simulink model "TST_EISGov_Governor"  (R2016b)
settings: Solver=FixedStepDiscrete  StartTime=0.0  StopTime=simTime  FixedStep=sampleTime  RelTol=1e-3
values from neighbouring files (symbols this model uses):
  testCase = 1    [initTST_EISGov_Governor_001.m]    (also in initTST_EISGov_Governor_002.m = 2; initTST_EISGov_Governor_003.m = 3; initTST_EISGov_Governor_004.m = 4; initTST_EISGov_Governor_005.m = 5)
libraries: simulink x43, UnitTest_Lib x36
(part 1 of 4)
settings Model: Creator=zhengjinyan  LastModifiedBy=zhengjinyan
settings DebuggingCC: SignalRangeChecking=error

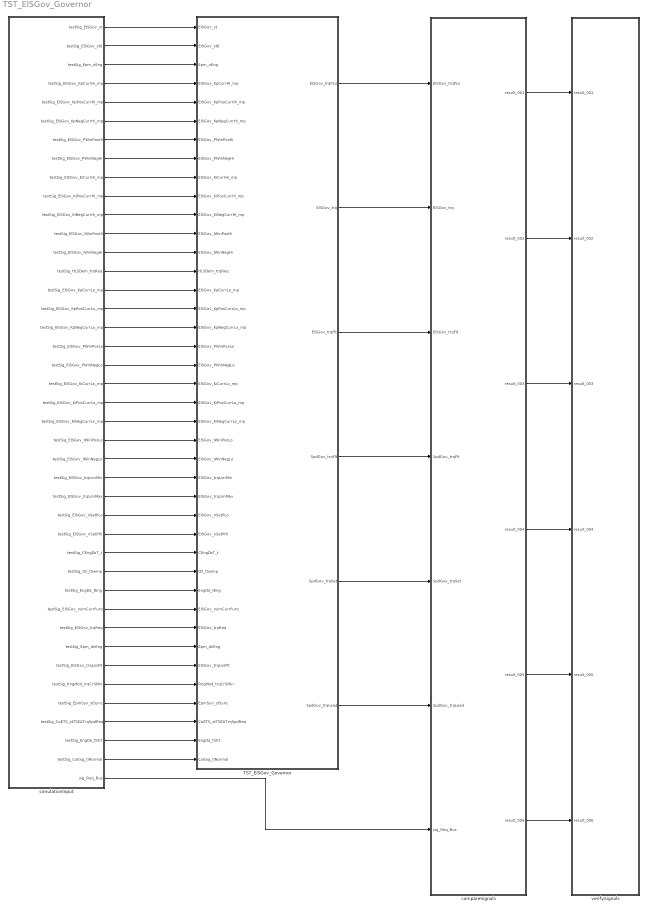
== system TST_EISGov_Governor ==
  TST_EISGov_Governor : Subsystem
  compareSignals : Subsystem
  simulationInput : Subsystem
  verifySignals : Subsystem
  wires:
  simulationInput/1(testSig_EISGov_st) -> TST_EISGov_Governor/1(EISGov_st)
  simulationInput/2(testSig_EISGov_st6) -> TST_EISGov_Governor/2(EISGov_st6)
  simulationInput/3(testSig_Epm_nEng) -> TST_EISGov_Governor/3(Epm_nEng)
  simulationInput/4(testSig_EISGov_KpCurrHi_mp) -> TST_EISGov_Governor/4(EISGov_KpCurrHi_mp)
  simulationInput/5(testSig_EISGov_KpPosCurrHi_mp) -> TST_EISGov_Governor/5(EISGov_KpPosCurrHi_mp)
  simulationInput/6(testSig_EISGov_KpNegCurrHi_mp) -> TST_EISGov_Governor/6(EISGov_KpNegCurrHi_mp)
  simulationInput/7(testSig_EISGov_PWinPosHi) -> TST_EISGov_Governor/7(EISGov_PWinPosHi)
  simulationInput/8(testSig_EISGov_PWinNegHi) -> TST_EISGov_Governor/8(EISGov_PWinNegHi)
  simulationInput/9(testSig_EISGov_KiCurrHi_mp) -> TST_EISGov_Governor/9(EISGov_KiCurrHi_mp)
  simulationInput/10(testSig_EISGov_KiPosCurrHi_mp) -> TST_EISGov_Governor/10(EISGov_KiPosCurrHi_mp)
  simulationInput/11(testSig_EISGov_KiNegCurrHi_mp) -> TST_EISGov_Governor/11(EISGov_KiNegCurrHi_mp)
  simulationInput/12(testSig_EISGov_IWinPosHi) -> TST_EISGov_Governor/12(EISGov_IWinPosHi)
  simulationInput/13(testSig_EISGov_IWinNegHi) -> TST_EISGov_Governor/13(EISGov_IWinNegHi)
  simulationInput/14(testSig_HLSDem_trqReq) -> TST_EISGov_Governor/14(HLSDem_trqReq)
  simulationInput/15(testSig_EISGov_KpCurrLo_mp) -> TST_EISGov_Governor/15(EISGov_KpCurrLo_mp)
  simulationInput/16(testSig_EISGov_KpPosCurrLo_mp) -> TST_EISGov_Governor/16(EISGov_KpPosCurrLo_mp)
  simulationInput/17(testSig_EISGov_KpNegCurrLo_mp) -> TST_EISGov_Governor/17(EISGov_KpNegCurrLo_mp)
  simulationInput/18(testSig_EISGov_PWinPosLo) -> TST_EISGov_Governor/18(EISGov_PWinPosLo)
  simulationInput/19(testSig_EISGov_PWinNegLo) -> TST_EISGov_Governor/19(EISGov_PWinNegLo)
  simulationInput/20(testSig_EISGov_KiCurrLo_mp) -> TST_EISGov_Governor/20(EISGov_KiCurrLo_mp)
  simulationInput/21(testSig_EISGov_KiPosCurrLo_mp) -> TST_EISGov_Governor/21(EISGov_KiPosCurrLo_mp)
  simulationInput/22(testSig_EISGov_KiNegCurrLo_mp) -> TST_EISGov_Governor/22(EISGov_KiNegCurrLo_mp)
  simulationInput/23(testSig_EISGov_IWinPosLo) -> TST_EISGov_Governor/23(EISGov_IWinPosLo)
  simulationInput/24(testSig_EISGov_IWinNegLo) -> TST_EISGov_Governor/24(EISGov_IWinNegLo)
  simulationInput/25(testSig_EISGov_trqLimMin) -> TST_EISGov_Governor/25(EISGov_trqLimMin)
  simulationInput/26(testSig_EISGov_trqLimMax) -> TST_EISGov_Governor/26(EISGov_trqLimMax)
  simulationInput/27(testSig_EISGov_nSetPLo) -> TST_EISGov_Governor/27(EISGov_nSetPLo)
  simulationInput/28(testSig_EISGov_nSetPHi) -> TST_EISGov_Governor/28(EISGov_nSetPHi)
  simulationInput/29(testSig_CEngDsT_t) -> TST_EISGov_Governor/29(CEngDsT_t)
  simulationInput/30(testSig_Oil_tSwmp) -> TST_EISGov_Governor/30(Oil_tSwmp)
  simulationInput/31(testSig_EngDa_tEng) -> TST_EISGov_Governor/31(EngDa_tEng)
  simulationInput/32(testSig_EISGov_numCurrFunc) -> TST_EISGov_Governor/32(EISGov_numCurrFunc)
  simulationInput/33(testSig_EISGov_trqReq) -> TST_EISGov_Governor/33(EISGov_trqReq)
  simulationInput/34(testSig_Epm_dnEng) -> TST_EISGov_Governor/34(Epm_dnEng)
  simulationInput/35(testSig_EISGov_trqLosFlt) -> TST_EISGov_Governor/35(EISGov_trqLosFlt)
  simulationInput/36(testSig_RngMod_trqCrSMin) -> TST_EISGov_Governor/36(RngMod_trqCrSMin)
  simulationInput/37(testSig_EpmSyn_stSync) -> TST_EISGov_Governor/37(EpmSyn_stSync)
  simulationInput/38(testSig_CoETS_stTSEATrqSpdReq) -> TST_EISGov_Governor/38(CoETS_stTSEATrqSpdReq)
  simulationInput/39(testSig_EngDa_tStrt) -> TST_EISGov_Governor/39(EngDa_tStrt)
  simulationInput/40(testSig_CoEng_tiNormal) -> TST_EISGov_Governor/40(CoEng_tiNormal)
  TST_EISGov_Governor/1(EISGov_trqPLo) -> compareSignals/1(EISGov_trqPLo)
  TST_EISGov_Governor/2(EISGov_trq) -> compareSignals/2(EISGov_trq)
  TST_EISGov_Governor/3(EISGov_trqFlt) -> compareSignals/3(EISGov_trqFlt)
  TST_EISGov_Governor/4(SpdGov_trqFlt) -> compareSignals/4(SpdGov_trqFlt)
  TST_EISGov_Governor/5(SpdGov_trqSet) -> compareSignals/5(SpdGov_trqSet)
  TST_EISGov_Governor/6(SpdGov_trqLead) -> compareSignals/6(SpdGov_trqLead)
  simulationInput/41(sig_Req_Bus) -> compareSignals/7(sig_Req_Bus)
  compareSignals/1(result_001) -> verifySignals/1(result_001)
  compareSignals/2(result_002) -> verifySignals/2(result_002)
  compareSignals/3(result_003) -> verifySignals/3(result_003)
  compareSignals/4(result_004) -> verifySignals/4(result_004)
  compareSignals/5(result_005) -> verifySignals/5(result_005)
  compareSignals/6(result_006) -> verifySignals/6(result_006)

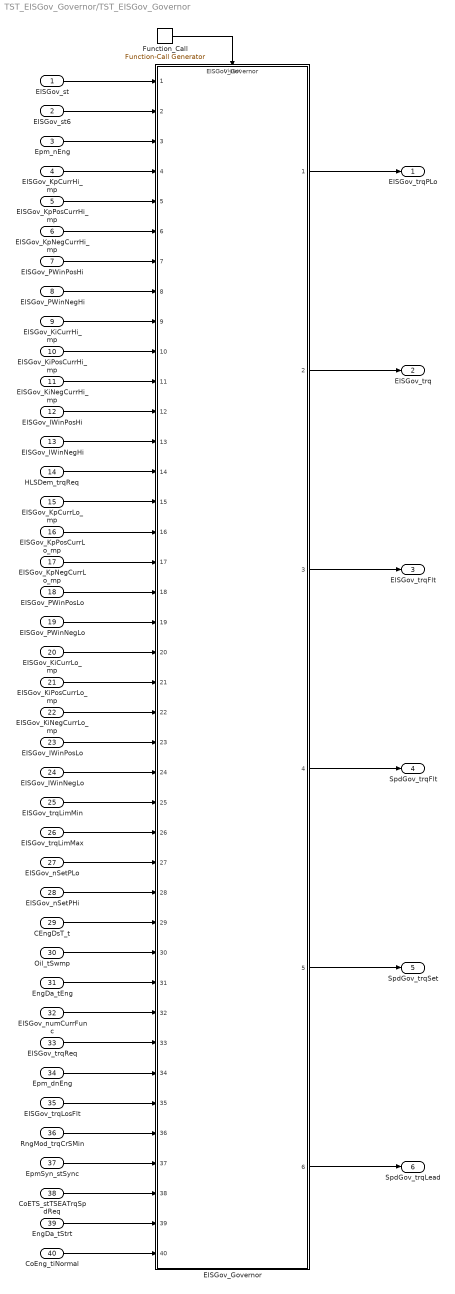
== system TST_EISGov_Governor/TST_EISGov_Governor ==
  EISGov_st : Inport
  EISGov_st6 : Inport  Port=2
  Epm_nEng : Inport  Port=3
  EISGov_KpCurrHi_mp : Inport  Port=4
  EISGov_KpPosCurrHi_mp : Inport  Port=5
  EISGov_KpNegCurrHi_mp : Inport  Port=6
  EISGov_PWinPosHi : Inport  Port=7
  EISGov_PWinNegHi : Inport  Port=8
  EISGov_KiCurrHi_mp : Inport  Port=9
  EISGov_KiPosCurrHi_mp : Inport  Port=10
  EISGov_KiNegCurrHi_mp : Inport  Port=11
  EISGov_IWinPosHi : Inport  Port=12
  EISGov_IWinNegHi : Inport  Port=13
  HLSDem_trqReq : Inport  Port=14
  EISGov_KpCurrLo_mp : Inport  Port=15
  EISGov_KpPosCurrLo_mp : Inport  Port=16
  EISGov_KpNegCurrLo_mp : Inport  Port=17
  EISGov_PWinPosLo : Inport  Port=18
  EISGov_PWinNegLo : Inport  Port=19
  EISGov_KiCurrLo_mp : Inport  Port=20
  EISGov_KiPosCurrLo_mp : Inport  Port=21
  EISGov_KiNegCurrLo_mp : Inport  Port=22
  EISGov_IWinPosLo : Inport  Port=23
  EISGov_IWinNegLo : Inport  Port=24
  EISGov_trqLimMin : Inport  Port=25
  EISGov_trqLimMax : Inport  Port=26
  EISGov_nSetPLo : Inport  Port=27
  EISGov_nSetPHi : Inport  Port=28
  CEngDsT_t : Inport  Port=29
  Oil_tSwmp : Inport  Port=30
  EngDa_tEng : Inport  Port=31
  EISGov_numCurrFunc : Inport  Port=32
  EISGov_trqReq : Inport  Port=33
  Epm_dnEng : Inport  Port=34
  EISGov_trqLosFlt : Inport  Port=35
  RngMod_trqCrSMin : Inport  Port=36
  EpmSyn_stSync : Inport  Port=37
  CoETS_stTSEATrqSpdReq : Inport  Port=38
  EngDa_tStrt : Inport  Port=39
  CoEng_tiNormal : Inport  Port=40
  EISGov_Governor : ModelReference  ModelNameDialog=EISGov_Governor  SimulationMode=Normal  ModelReferenceVersion=1.324  TriggerPortName=function  TriggerPortTriggerType=function-call  TriggerPortStatesWhenEnabling=held
  Function_Call : simulink/Ports & Subsystems/Function-Call Generator  sample_time=sampleTime  numberOfIterations=1
  EISGov_trqPLo : Outport
  EISGov_trq : Outport  Port=2
  EISGov_trqFlt : Outport  Port=3
  SpdGov_trqFlt : Outport  Port=4
  SpdGov_trqSet : Outport  Port=5
  SpdGov_trqLead : Outport  Port=6
  wires:
  Function_Call/1 -> EISGov_Governor/Trigger
  EISGov_st/1 -> EISGov_Governor/1
  EISGov_st6/1 -> EISGov_Governor/2
  Epm_nEng/1 -> EISGov_Governor/3
  EISGov_KpCurrHi_mp/1 -> EISGov_Governor/4
  EISGov_KpPosCurrHi_mp/1 -> EISGov_Governor/5
  EISGov_KpNegCurrHi_mp/1 -> EISGov_Governor/6
  EISGov_PWinPosHi/1 -> EISGov_Governor/7
  EISGov_PWinNegHi/1 -> EISGov_Governor/8
  EISGov_KiCurrHi_mp/1 -> EISGov_Governor/9
  EISGov_KiPosCurrHi_mp/1 -> EISGov_Governor/10
  EISGov_KiNegCurrHi_mp/1 -> EISGov_Governor/11
  EISGov_IWinPosHi/1 -> EISGov_Governor/12
  EISGov_IWinNegHi/1 -> EISGov_Governor/13
  HLSDem_trqReq/1 -> EISGov_Governor/14
  EISGov_KpCurrLo_mp/1 -> EISGov_Governor/15
  EISGov_KpPosCurrLo_mp/1 -> EISGov_Governor/16
  EISGov_KpNegCurrLo_mp/1 -> EISGov_Governor/17
  EISGov_PWinPosLo/1 -> EISGov_Governor/18
  EISGov_PWinNegLo/1 -> EISGov_Governor/19
  EISGov_KiCurrLo_mp/1 -> EISGov_Governor/20
  EISGov_KiPosCurrLo_mp/1 -> EISGov_Governor/21
  EISGov_KiNegCurrLo_mp/1 -> EISGov_Governor/22
  EISGov_IWinPosLo/1 -> EISGov_Governor/23
  EISGov_IWinNegLo/1 -> EISGov_Governor/24
  EISGov_trqLimMin/1 -> EISGov_Governor/25
  EISGov_trqLimMax/1 -> EISGov_Governor/26
  EISGov_nSetPLo/1 -> EISGov_Governor/27
  EISGov_nSetPHi/1 -> EISGov_Governor/28
  CEngDsT_t/1 -> EISGov_Governor/29
  Oil_tSwmp/1 -> EISGov_Governor/30
  EngDa_tEng/1 -> EISGov_Governor/31
  EISGov_numCurrFunc/1 -> EISGov_Governor/32
  EISGov_trqReq/1 -> EISGov_Governor/33
  Epm_dnEng/1 -> EISGov_Governor/34
  EISGov_trqLosFlt/1 -> EISGov_Governor/35
  RngMod_trqCrSMin/1 -> EISGov_Governor/36
  EpmSyn_stSync/1 -> EISGov_Governor/37
  CoETS_stTSEATrqSpdReq/1 -> EISGov_Governor/38
  EngDa_tStrt/1 -> EISGov_Governor/39
  CoEng_tiNormal/1 -> EISGov_Governor/40
  EISGov_Governor/1 -> EISGov_trqPLo/1
  EISGov_Governor/2 -> EISGov_trq/1
  EISGov_Governor/3 -> EISGov_trqFlt/1
  EISGov_Governor/4 -> SpdGov_trqFlt/1
  EISGov_Governor/5 -> SpdGov_trqSet/1
  EISGov_Governor/6 -> SpdGov_trqLead/1

== system TST_EISGov_Governor/compareSignals ==
  EISGov_trqPLo : Inport
  EISGov_trq : Inport  Port=2
  EISGov_trqFlt : Inport  Port=3
  SpdGov_trqFlt : Inport  Port=4
  SpdGov_trqSet : Inport  Port=5
  SpdGov_trqLead : Inport  Port=6
  sig_Req_Bus : Inport  Port=7
  BC : BusCreator  Inputs=6
  CTC_001 : simulink/Logic and Bit Operations/Compare To Constant  relop===  const=1  OutDataTypeStr=boolean
  CTC_002 : simulink/Logic and Bit Operations/Compare To Constant  relop===  const=2  OutDataTypeStr=boolean
  CTC_003 : simulink/Logic and Bit Operations/Compare To Constant  relop===  const=3  OutDataTypeStr=boolean
  CTC_004 : simulink/Logic and Bit Operations/Compare To Constant  relop===  const=4  OutDataTypeStr=boolean
  CTC_005 : simulink/Logic and Bit Operations/Compare To Constant  relop===  const=5  OutDataTypeStr=boolean
  CTC_006 : simulink/Logic and Bit Operations/Compare To Constant  relop===  const=6  OutDataTypeStr=boolean
  Requirement_001 : Subsystem
  Requirement_002 : Subsystem
  Requirement_003 : Subsystem
  Requirement_004 : Subsystem
  Requirement_005 : Subsystem
  Requirement_006 : Subsystem
  TC_001 : Constant  Value=testCase
  TC_002 : Constant  Value=testCase
  TC_003 : Constant  Value=testCase
  TC_004 : Constant  Value=testCase
  TC_005 : Constant  Value=testCase
  TC_006 : Constant  Value=testCase
  result_001 : Outport
  result_002 : Outport  Port=2
  result_003 : Outport  Port=3
  result_004 : Outport  Port=4
  result_005 : Outport  Port=5
  result_006 : Outport  Port=6
  wires:
  EISGov_trqPLo/1 -> BC/1  "EISGov_trqPLo"
  EISGov_trq/1 -> BC/2  "EISGov_trq"
  EISGov_trqFlt/1 -> BC/3  "EISGov_trqFlt"
  SpdGov_trqFlt/1 -> BC/4  "SpdGov_trqFlt"
  SpdGov_trqSet/1 -> BC/5  "SpdGov_trqSet"
  SpdGov_trqLead/1 -> BC/6  "SpdGov_trqLead"
  TC_001/1 -> CTC_001/1
  CTC_001/1 -> Requirement_001/Enable
  sig_Req_Bus/1 -> Requirement_001/2(sig_Req_Bus), Requirement_002/2(sig_Req_Bus), Requirement_003/2(sig_Req_Bus), Requirement_004/2(sig_Req_Bus), Requirement_005/2(sig_Req_Bus), Requirement_006/2(sig_Req_Bus)
  BC/1 -> Requirement_001/1(sig_Result_Bus), Requirement_002/1(sig_Result_Bus), Requirement_003/1(sig_Result_Bus), Requirement_004/1(sig_Result_Bus), Requirement_005/1(sig_Result_Bus), Requirement_006/1(sig_Result_Bus)
  Requirement_001/1(result) -> result_001/1
  TC_002/1 -> CTC_002/1
  CTC_002/1 -> Requirement_002/Enable
  Requirement_002/1(result) -> result_002/1
  TC_003/1 -> CTC_003/1
  CTC_003/1 -> Requirement_003/Enable
  Requirement_003/1(result) -> result_003/1
  TC_004/1 -> CTC_004/1
  CTC_004/1 -> Requirement_004/Enable
  Requirement_004/1(result) -> result_004/1
  TC_005/1 -> CTC_005/1
  CTC_005/1 -> Requirement_005/Enable
  Requirement_005/1(result) -> result_005/1
  TC_006/1 -> CTC_006/1
  CTC_006/1 -> Requirement_006/Enable
  Requirement_006/1(result) -> result_006/1

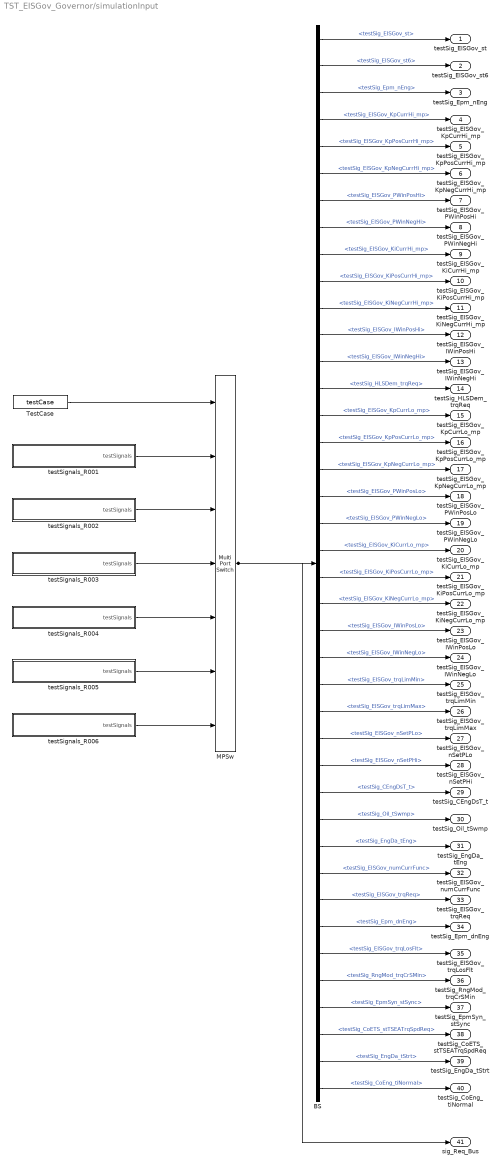
== system TST_EISGov_Governor/simulationInput ==
  BS : BusSelector  OutputSignals=testSig_EISGov_st,testSig_EISGov_st6,testSig_Epm_nEng,testSig_EISGov_KpCurrHi_mp,testSig_EISGov_KpPosCurrHi_mp,testSig_EISGov_KpNegCurrHi_mp,testSig_EISGov_PWinPosHi,testSig_EISGov_PWinNegHi,testSig_EISGov_KiCurrHi_mp,testSig_EISGov_KiPosCurrHi_mp,testSig_EISGov_KiNegCurrHi_mp,testSig_EISGov_IWinPosHi,testSig_EISGov_IWinNegHi,testSig_HLSDem_trqReq,testSig_EISGov_KpCurrLo_mp,testSig_EISGov_KpPosCurrLo_mp,testSig_EISGov_KpNegCurrLo_mp,testSig_EISGov_PWinPosLo,testSig_EISGov_PWinNegLo,testSig_EISGov_KiCurrLo_mp,testSig_EISGov_KiPosCurrLo_mp,testSig_EISGov_KiNegCurrLo_mp,testSig_EISGov_IWinPosLo,testSig_EISGov_IWinNegLo,testSig_EISGov_trqLimMin,testSig_EISGov_trqLimMax,testSig_EISGov_nSetPLo,testSig_EISGov_nSetPHi,testSig_CEngDsT_t,testSig_Oil_tSwmp,testSig_EngDa_tEng,testSig_EISGov_numCurrFunc,testSig_EISGov_trqReq,testSig_Epm_dnEng,testSig_EISGov_trqLosFlt,testSig_RngMod_trqCrSMin,testSig_EpmSyn_stSync,testSig_CoETS_stTSEATrqSpdReq,testSig_EngDa_tStrt,testSig_CoEng_tiNormal
  MPSw : MultiPortSwitch  Inputs=6  SaturateOnIntegerOverflow=on  InputSameDT=on
  TestCase : Constant  Value=testCase
  testSignals_R001 : Subsystem
  testSignals_R002 : Subsystem
  testSignals_R003 : Subsystem
  testSignals_R004 : Subsystem
  testSignals_R005 : Subsystem
  testSignals_R006 : Subsystem
  testSig_EISGov_st : Outport
  testSig_EISGov_st6 : Outport  Port=2
  testSig_Epm_nEng : Outport  Port=3
  testSig_EISGov_KpCurrHi_mp : Outport  Port=4
  testSig_EISGov_KpPosCurrHi_mp : Outport  Port=5
  testSig_EISGov_KpNegCurrHi_mp : Outport  Port=6
  testSig_EISGov_PWinPosHi : Outport  Port=7
  testSig_EISGov_PWinNegHi : Outport  Port=8
  testSig_EISGov_KiCurrHi_mp : Outport  Port=9
  testSig_EISGov_KiPosCurrHi_mp : Outport  Port=10
  testSig_EISGov_KiNegCurrHi_mp : Outport  Port=11
  testSig_EISGov_IWinPosHi : Outport  Port=12
  testSig_EISGov_IWinNegHi : Outport  Port=13
  testSig_HLSDem_trqReq : Outport  Port=14
  testSig_EISGov_KpCurrLo_mp : Outport  Port=15
  testSig_EISGov_KpPosCurrLo_mp : Outport  Port=16
  testSig_EISGov_KpNegCurrLo_mp : Outport  Port=17
  testSig_EISGov_PWinPosLo : Outport  Port=18
  testSig_EISGov_PWinNegLo : Outport  Port=19
  testSig_EISGov_KiCurrLo_mp : Outport  Port=20
  testSig_EISGov_KiPosCurrLo_mp : Outport  Port=21
  testSig_EISGov_KiNegCurrLo_mp : Outport  Port=22
  testSig_EISGov_IWinPosLo : Outport  Port=23
  testSig_EISGov_IWinNegLo : Outport  Port=24
  testSig_EISGov_trqLimMin : Outport  Port=25
  testSig_EISGov_trqLimMax : Outport  Port=26
  testSig_EISGov_nSetPLo : Outport  Port=27
  testSig_EISGov_nSetPHi : Outport  Port=28
  testSig_CEngDsT_t : Outport  Port=29
  testSig_Oil_tSwmp : Outport  Port=30
  testSig_EngDa_tEng : Outport  Port=31
  testSig_EISGov_numCurrFunc : Outport  Port=32
  testSig_EISGov_trqReq : Outport  Port=33
  testSig_Epm_dnEng : Outport  Port=34
  testSig_EISGov_trqLosFlt : Outport  Port=35
  testSig_RngMod_trqCrSMin : Outport  Port=36
  testSig_EpmSyn_stSync : Outport  Port=37
  testSig_CoETS_stTSEATrqSpdReq : Outport  Port=38
  testSig_EngDa_tStrt : Outport  Port=39
  testSig_CoEng_tiNormal : Outport  Port=40
  sig_Req_Bus : Outport  Port=41
  wires:
  BS/1 -> testSig_EISGov_st/1  "<testSig_EISGov_st>"
  BS/2 -> testSig_EISGov_st6/1  "<testSig_EISGov_st6>"
  BS/3 -> testSig_Epm_nEng/1  "<testSig_Epm_nEng>"
  BS/4 -> testSig_EISGov_KpCurrHi_mp/1  "<testSig_EISGov_KpCurrHi_mp>"
  BS/5 -> testSig_EISGov_KpPosCurrHi_mp/1  "<testSig_EISGov_KpPosCurrHi_mp>"
  BS/6 -> testSig_EISGov_KpNegCurrHi_mp/1  "<testSig_EISGov_KpNegCurrHi_mp>"
  BS/7 -> testSig_EISGov_PWinPosHi/1  "<testSig_EISGov_PWinPosHi>"
  BS/8 -> testSig_EISGov_PWinNegHi/1  "<testSig_EISGov_PWinNegHi>"
  BS/9 -> testSig_EISGov_KiCurrHi_mp/1  "<testSig_EISGov_KiCurrHi_mp>"
  BS/10 -> testSig_EISGov_KiPosCurrHi_mp/1  "<testSig_EISGov_KiPosCurrHi_mp>"
  BS/11 -> testSig_EISGov_KiNegCurrHi_mp/1  "<testSig_EISGov_KiNegCurrHi_mp>"
  BS/12 -> testSig_EISGov_IWinPosHi/1  "<testSig_EISGov_IWinPosHi>"
  BS/13 -> testSig_EISGov_IWinNegHi/1  "<testSig_EISGov_IWinNegHi>"
  BS/14 -> testSig_HLSDem_trqReq/1  "<testSig_HLSDem_trqReq>"
  BS/15 -> testSig_EISGov_KpCurrLo_mp/1  "<testSig_EISGov_KpCurrLo_mp>"
  BS/16 -> testSig_EISGov_KpPosCurrLo_mp/1  "<testSig_EISGov_KpPosCurrLo_mp>"
  BS/17 -> testSig_EISGov_KpNegCurrLo_mp/1  "<testSig_EISGov_KpNegCurrLo_mp>"
  BS/18 -> testSig_EISGov_PWinPosLo/1  "<testSig_EISGov_PWinPosLo>"
  BS/19 -> testSig_EISGov_PWinNegLo/1  "<testSig_EISGov_PWinNegLo>"
  BS/20 -> testSig_EISGov_KiCurrLo_mp/1  "<testSig_EISGov_KiCurrLo_mp>"
  BS/21 -> testSig_EISGov_KiPosCurrLo_mp/1  "<testSig_EISGov_KiPosCurrLo_mp>"
  BS/22 -> testSig_EISGov_KiNegCurrLo_mp/1  "<testSig_EISGov_KiNegCurrLo_mp>"
  BS/23 -> testSig_EISGov_IWinPosLo/1  "<testSig_EISGov_IWinPosLo>"
  BS/24 -> testSig_EISGov_IWinNegLo/1  "<testSig_EISGov_IWinNegLo>"
  BS/25 -> testSig_EISGov_trqLimMin/1  "<testSig_EISGov_trqLimMin>"
  BS/26 -> testSig_EISGov_trqLimMax/1  "<testSig_EISGov_trqLimMax>"
  BS/27 -> testSig_EISGov_nSetPLo/1  "<testSig_EISGov_nSetPLo>"
  BS/28 -> testSig_EISGov_nSetPHi/1  "<testSig_EISGov_nSetPHi>"
  BS/29 -> testSig_CEngDsT_t/1  "<testSig_CEngDsT_t>"
  BS/30 -> testSig_Oil_tSwmp/1  "<testSig_Oil_tSwmp>"
  BS/31 -> testSig_EngDa_tEng/1  "<testSig_EngDa_tEng>"
  BS/32 -> testSig_EISGov_numCurrFunc/1  "<testSig_EISGov_numCurrFunc>"
  BS/33 -> testSig_EISGov_trqReq/1  "<testSig_EISGov_trqReq>"
  BS/34 -> testSig_Epm_dnEng/1  "<testSig_Epm_dnEng>"
  BS/35 -> testSig_EISGov_trqLosFlt/1  "<testSig_EISGov_trqLosFlt>"
  BS/36 -> testSig_RngMod_trqCrSMin/1  "<testSig_RngMod_trqCrSMin>"
  BS/37 -> testSig_EpmSyn_stSync/1  "<testSig_EpmSyn_stSync>"
  BS/38 -> testSig_CoETS_stTSEATrqSpdReq/1  "<testSig_CoETS_stTSEATrqSpdReq>"
  BS/39 -> testSig_EngDa_tStrt/1  "<testSig_EngDa_tStrt>"
  BS/40 -> testSig_CoEng_tiNormal/1  "<testSig_CoEng_tiNormal>"
  MPSw/1 -> BS/1, sig_Req_Bus/1
  TestCase/1 -> MPSw/1
  testSignals_R001/1(testSignals) -> MPSw/2
  testSignals_R002/1(testSignals) -> MPSw/3
  testSignals_R003/1(testSignals) -> MPSw/4
  testSignals_R004/1(testSignals) -> MPSw/5
  testSignals_R005/1(testSignals) -> MPSw/6
  testSignals_R006/1(testSignals) -> MPSw/7

== system TST_EISGov_Governor/verifySignals ==
  result_001 : Inport
  result_002 : Inport  Port=2
  result_003 : Inport  Port=3
  result_004 : Inport  Port=4
  result_005 : Inport  Port=5
  result_006 : Inport  Port=6
  Assertion_001 : Assertion  Enabled=off
  Assertion_002 : Assertion  Enabled=off
  Assertion_003 : Assertion  Enabled=off
  Assertion_004 : Assertion  Enabled=off
  Assertion_005 : Assertion  Enabled=off
  Assertion_006 : Assertion  Enabled=off
  wires:
  result_001/1 -> Assertion_001/1
  result_002/1 -> Assertion_002/1
  result_003/1 -> Assertion_003/1
  result_004/1 -> Assertion_004/1
  result_005/1 -> Assertion_005/1
  result_006/1 -> Assertion_006/1

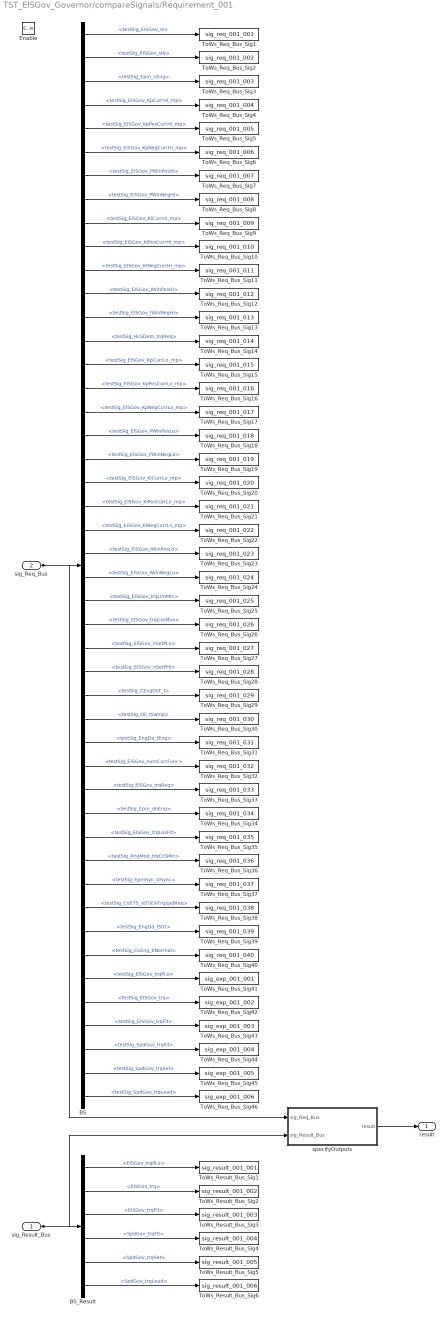
== system TST_EISGov_Governor/compareSignals/Requirement_001 ==
  sig_Result_Bus : Inport
  sig_Req_Bus : Inport  Port=2
  Enable : EnablePort
  BS : BusSelector  OutputSignals=testSig_EISGov_st,testSig_EISGov_st6,testSig_Epm_nEng,testSig_EISGov_KpCurrHi_mp,testSig_EISGov_KpPosCurrHi_mp,testSig_EISGov_KpNegCurrHi_mp,testSig_EISGov_PWinPosHi,testSig_EISGov_PWinNegHi,testSig_EISGov_KiCurrHi_mp,testSig_EISGov_KiPosCurrHi_mp,testSig_EISGov_KiNegCurrHi_mp,testSig_EISGov_IWinPosHi,testSig_EISGov_IWinNegHi,testSig_HLSDem_trqReq,testSig_EISGov_KpCurrLo_mp,testSig_EISGov_KpPosCurrLo_mp,testSig_EISGov_KpNegCurrLo_mp,testSig_EISGov_PWinPosLo,testSig_EISGov_PWinNegLo,testSig_EISGov_KiCurrLo_mp,testSig_EISGov_KiPosCurrLo_mp,testSig_EISGov_KiNegCurrLo_mp,testSig_EISGov_IWinPosLo,testSig_EISGov_IWinNegLo,testSig_EISGov_trqLimMin,testSig_EISGov_trqLimMax,testSig_EISGov_nSetPLo,testSig_EISGov_nSetPHi,testSig_CEngDsT_t,testSig_Oil_tSwmp,testSig_EngDa_tEng,testSig_EISGov_numCurrFunc,testSig_EISGov_trqReq,testSig_Epm_dnEng,testSig_EISGov_trqLosFlt,testSig_RngMod_trqCrSMin,testSig_EpmSyn_stSync,testSig_CoETS_stTSEATrqSpdReq,testSig_EngDa_tStrt,testSig_CoEng_tiNormal,testSig_EISGov_trqPLo,testSig_EISGov_trq,testSig_EISGov_trqFlt,testSig_SpdGov_trqFlt,testSig_SpdGov_trqSet,testSig_SpdGov_trqLead
  BS_Result : BusSelector  OutputSignals=EISGov_trqPLo,EISGov_trq,EISGov_trqFlt,SpdGov_trqFlt,SpdGov_trqSet,SpdGov_trqLead
  ToWs_Req_Bus_Sig1 : ToWorkspace  VariableName=sig_req_001_001  SaveFormat=Structure With Time
  ToWs_Req_Bus_Sig10 : ToWorkspace  VariableName=sig_req_001_010  SaveFormat=Structure With Time
  ToWs_Req_Bus_Sig11 : ToWorkspace  VariableName=sig_req_001_011  SaveFormat=Structure With Time
  ToWs_Req_Bus_Sig12 : ToWorkspace  VariableName=sig_req_001_012  SaveFormat=Structure With Time
  ToWs_Req_Bus_Sig13 : ToWorkspace  VariableName=sig_req_001_013  SaveFormat=Structure With Time
  ToWs_Req_Bus_Sig14 : ToWorkspace  VariableName=sig_req_001_014  SaveFormat=Structure With Time
  ToWs_Req_Bus_Sig15 : ToWorkspace  VariableName=sig_req_001_015  SaveFormat=Structure With Time
  ToWs_Req_Bus_Sig16 : ToWorkspace  VariableName=sig_req_001_016  SaveFormat=Structure With Time
  ToWs_Req_Bus_Sig17 : ToWorkspace  VariableName=sig_req_001_017  SaveFormat=Structure With Time
  ToWs_Req_Bus_Sig18 : ToWorkspace  VariableName=sig_req_001_018  SaveFormat=Structure With Time
  ToWs_Req_Bus_Sig19 : ToWorkspace  VariableName=sig_req_001_019  SaveFormat=Structure With Time
  ToWs_Req_Bus_Sig2 : ToWorkspace  VariableName=sig_req_001_002  SaveFormat=Structure With Time
  ToWs_Req_Bus_Sig20 : ToWorkspace  VariableName=sig_req_001_020  SaveFormat=Structure With Time
  ToWs_Req_Bus_Sig21 : ToWorkspace  VariableName=sig_req_001_021  SaveFormat=Structure With Time
  ToWs_Req_Bus_Sig22 : ToWorkspace  VariableName=sig_req_001_022  SaveFormat=Structure With Time
  ToWs_Req_Bus_Sig23 : ToWorkspace  VariableName=sig_req_001_023  SaveFormat=Structure With Time
  ToWs_Req_Bus_Sig24 : ToWorkspace  VariableName=sig_req_001_024  SaveFormat=Structure With Time
  ToWs_Req_Bus_Sig25 : ToWorkspace  VariableName=sig_req_001_025  SaveFormat=Structure With Time
  ToWs_Req_Bus_Sig26 : ToWorkspace  VariableName=sig_req_001_026  SaveFormat=Structure With Time
  ToWs_Req_Bus_Sig27 : ToWorkspace  VariableName=sig_req_001_027  SaveFormat=Structure With Time
  ToWs_Req_Bus_Sig28 : ToWorkspace  VariableName=sig_req_001_028  SaveFormat=Structure With Time
  ToWs_Req_Bus_Sig29 : ToWorkspace  VariableName=sig_req_001_029  SaveFormat=Structure With Time
  ToWs_Req_Bus_Sig3 : ToWorkspace  VariableName=sig_req_001_003  SaveFormat=Structure With Time
  ToWs_Req_Bus_Sig30 : ToWorkspace  VariableName=sig_req_001_030  SaveFormat=Structure With Time
  ToWs_Req_Bus_Sig31 : ToWorkspace  VariableName=sig_req_001_031  SaveFormat=Structure With Time
  ToWs_Req_Bus_Sig32 : ToWorkspace  VariableName=sig_req_001_032  SaveFormat=Structure With Time
  ToWs_Req_Bus_Sig33 : ToWorkspace  VariableName=sig_req_001_033  SaveFormat=Structure With Time
  ToWs_Req_Bus_Sig34 : ToWorkspace  VariableName=sig_req_001_034  SaveFormat=Structure With Time
  ToWs_Req_Bus_Sig35 : ToWorkspace  VariableName=sig_req_001_035  SaveFormat=Structure With Time
  ToWs_Req_Bus_Sig36 : ToWorkspace  VariableName=sig_req_001_036  SaveFormat=Structure With Time
  ToWs_Req_Bus_Sig37 : ToWorkspace  VariableName=sig_req_001_037  SaveFormat=Structure With Time
  ToWs_Req_Bus_Sig38 : ToWorkspace  VariableName=sig_req_001_038  SaveFormat=Structure With Time
  ToWs_Req_Bus_Sig39 : ToWorkspace  VariableName=sig_req_001_039  SaveFormat=Structure With Time
  ToWs_Req_Bus_Sig4 : ToWorkspace  VariableName=sig_req_001_004  SaveFormat=Structure With Time
  ToWs_Req_Bus_Sig40 : ToWorkspace  VariableName=sig_req_001_040  SaveFormat=Structure With Time
  ToWs_Req_Bus_Sig41 : ToWorkspace  VariableName=sig_exp_001_001  SaveFormat=Structure With Time
  ToWs_Req_Bus_Sig42 : ToWorkspace  VariableName=sig_exp_001_002  SaveFormat=Structure With Time
  ToWs_Req_Bus_Sig43 : ToWorkspace  VariableName=sig_exp_001_003  SaveFormat=Structure With Time
  ToWs_Req_Bus_Sig44 : ToWorkspace  VariableName=sig_exp_001_004  SaveFormat=Structure With Time
  ToWs_Req_Bus_Sig45 : ToWorkspace  VariableName=sig_exp_001_005  SaveFormat=Structure With Time
  ToWs_Req_Bus_Sig46 : ToWorkspace  VariableName=sig_exp_001_006  SaveFormat=Structure With Time
  ToWs_Req_Bus_Sig5 : ToWorkspace  VariableName=sig_req_001_005  SaveFormat=Structure With Time
  ToWs_Req_Bus_Sig6 : ToWorkspace  VariableName=sig_req_001_006  SaveFormat=Structure With Time
  ToWs_Req_Bus_Sig7 : ToWorkspace  VariableName=sig_req_001_007  SaveFormat=Structure With Time
  ToWs_Req_Bus_Sig8 : ToWorkspace  VariableName=sig_req_001_008  SaveFormat=Structure With Time
  ToWs_Req_Bus_Sig9 : ToWorkspace  VariableName=sig_req_001_009  SaveFormat=Structure With Time
  ToWs_Result_Bus_Sig1 : ToWorkspace  VariableName=sig_result_001_001  SaveFormat=Structure With Time
  ToWs_Result_Bus_Sig2 : ToWorkspace  VariableName=sig_result_001_002  SaveFormat=Structure With Time
  ToWs_Result_Bus_Sig3 : ToWorkspace  VariableName=sig_result_001_003  SaveFormat=Structure With Time
  ToWs_Result_Bus_Sig4 : ToWorkspace  VariableName=sig_result_001_004  SaveFormat=Structure With Time
  ToWs_Result_Bus_Sig5 : ToWorkspace  VariableName=sig_result_001_005  SaveFormat=Structure With Time
  ToWs_Result_Bus_Sig6 : ToWorkspace  VariableName=sig_result_001_006  SaveFormat=Structure With Time
  specifyOutputs : Subsystem
  result : Outport
  wires:
  sig_Req_Bus/1 -> BS/1, specifyOutputs/1(sig_Req_Bus)
  BS/1 -> ToWs_Req_Bus_Sig1/1  "<testSig_EISGov_st>"
  BS/2 -> ToWs_Req_Bus_Sig2/1  "<testSig_EISGov_st6>"
  BS/3 -> ToWs_Req_Bus_Sig3/1  "<testSig_Epm_nEng>"
  BS/4 -> ToWs_Req_Bus_Sig4/1  "<testSig_EISGov_KpCurrHi_mp>"
  BS/5 -> ToWs_Req_Bus_Sig5/1  "<testSig_EISGov_KpPosCurrHi_mp>"
  BS/6 -> ToWs_Req_Bus_Sig6/1  "<testSig_EISGov_KpNegCurrHi_mp>"
  BS/7 -> ToWs_Req_Bus_Sig7/1  "<testSig_EISGov_PWinPosHi>"
  BS/8 -> ToWs_Req_Bus_Sig8/1  "<testSig_EISGov_PWinNegHi>"
  BS/9 -> ToWs_Req_Bus_Sig9/1  "<testSig_EISGov_KiCurrHi_mp>"
  BS/10 -> ToWs_Req_Bus_Sig10/1  "<testSig_EISGov_KiPosCurrHi_mp>"
  BS/11 -> ToWs_Req_Bus_Sig11/1  "<testSig_EISGov_KiNegCurrHi_mp>"
  BS/12 -> ToWs_Req_Bus_Sig12/1  "<testSig_EISGov_IWinPosHi>"
  BS/13 -> ToWs_Req_Bus_Sig13/1  "<testSig_EISGov_IWinNegHi>"
  BS/14 -> ToWs_Req_Bus_Sig14/1  "<testSig_HLSDem_trqReq>"
  BS/15 -> ToWs_Req_Bus_Sig15/1  "<testSig_EISGov_KpCurrLo_mp>"
  BS/16 -> ToWs_Req_Bus_Sig16/1  "<testSig_EISGov_KpPosCurrLo_mp>"
  BS/17 -> ToWs_Req_Bus_Sig17/1  "<testSig_EISGov_KpNegCurrLo_mp>"
  BS/18 -> ToWs_Req_Bus_Sig18/1  "<testSig_EISGov_PWinPosLo>"
  BS/19 -> ToWs_Req_Bus_Sig19/1  "<testSig_EISGov_PWinNegLo>"
  BS/20 -> ToWs_Req_Bus_Sig20/1  "<testSig_EISGov_KiCurrLo_mp>"
  BS/21 -> ToWs_Req_Bus_Sig21/1  "<testSig_EISGov_KiPosCurrLo_mp>"
  BS/22 -> ToWs_Req_Bus_Sig22/1  "<testSig_EISGov_KiNegCurrLo_mp>"
  BS/23 -> ToWs_Req_Bus_Sig23/1  "<testSig_EISGov_IWinPosLo>"
  BS/24 -> ToWs_Req_Bus_Sig24/1  "<testSig_EISGov_IWinNegLo>"
  BS/25 -> ToWs_Req_Bus_Sig25/1  "<testSig_EISGov_trqLimMin>"
  BS/26 -> ToWs_Req_Bus_Sig26/1  "<testSig_EISGov_trqLimMax>"
  BS/27 -> ToWs_Req_Bus_Sig27/1  "<testSig_EISGov_nSetPLo>"
  BS/28 -> ToWs_Req_Bus_Sig28/1  "<testSig_EISGov_nSetPHi>"
  BS/29 -> ToWs_Req_Bus_Sig29/1  "<testSig_CEngDsT_t>"
  BS/30 -> ToWs_Req_Bus_Sig30/1  "<testSig_Oil_tSwmp>"
  BS/31 -> ToWs_Req_Bus_Sig31/1  "<testSig_EngDa_tEng>"
  BS/32 -> ToWs_Req_Bus_Sig32/1  "<testSig_EISGov_numCurrFunc>"
  BS/33 -> ToWs_Req_Bus_Sig33/1  "<testSig_EISGov_trqReq>"
  BS/34 -> ToWs_Req_Bus_Sig34/1  "<testSig_Epm_dnEng>"
  BS/35 -> ToWs_Req_Bus_Sig35/1  "<testSig_EISGov_trqLosFlt>"
  BS/36 -> ToWs_Req_Bus_Sig36/1  "<testSig_RngMod_trqCrSMin>"
  BS/37 -> ToWs_Req_Bus_Sig37/1  "<testSig_EpmSyn_stSync>"
  BS/38 -> ToWs_Req_Bus_Sig38/1  "<testSig_CoETS_stTSEATrqSpdReq>"
  BS/39 -> ToWs_Req_Bus_Sig39/1  "<testSig_EngDa_tStrt>"
  BS/40 -> ToWs_Req_Bus_Sig40/1  "<testSig_CoEng_tiNormal>"
  BS/41 -> ToWs_Req_Bus_Sig41/1  "<testSig_EISGov_trqPLo>"
  BS/42 -> ToWs_Req_Bus_Sig42/1  "<testSig_EISGov_trq>"
  BS/43 -> ToWs_Req_Bus_Sig43/1  "<testSig_EISGov_trqFlt>"
  BS/44 -> ToWs_Req_Bus_Sig44/1  "<testSig_SpdGov_trqFlt>"
  BS/45 -> ToWs_Req_Bus_Sig45/1  "<testSig_SpdGov_trqSet>"
  BS/46 -> ToWs_Req_Bus_Sig46/1  "<testSig_SpdGov_trqLead>"
  sig_Result_Bus/1 -> BS_Result/1, specifyOutputs/2(sig_Result_Bus)
  BS_Result/1 -> ToWs_Result_Bus_Sig1/1  "<EISGov_trqPLo>"
  BS_Result/2 -> ToWs_Result_Bus_Sig2/1  "<EISGov_trq>"
  BS_Result/3 -> ToWs_Result_Bus_Sig3/1  "<EISGov_trqFlt>"
  BS_Result/4 -> ToWs_Result_Bus_Sig4/1  "<SpdGov_trqFlt>"
  BS_Result/5 -> ToWs_Result_Bus_Sig5/1  "<SpdGov_trqSet>"
  BS_Result/6 -> ToWs_Result_Bus_Sig6/1  "<SpdGov_trqLead>"
  specifyOutputs/1(result) -> result/1

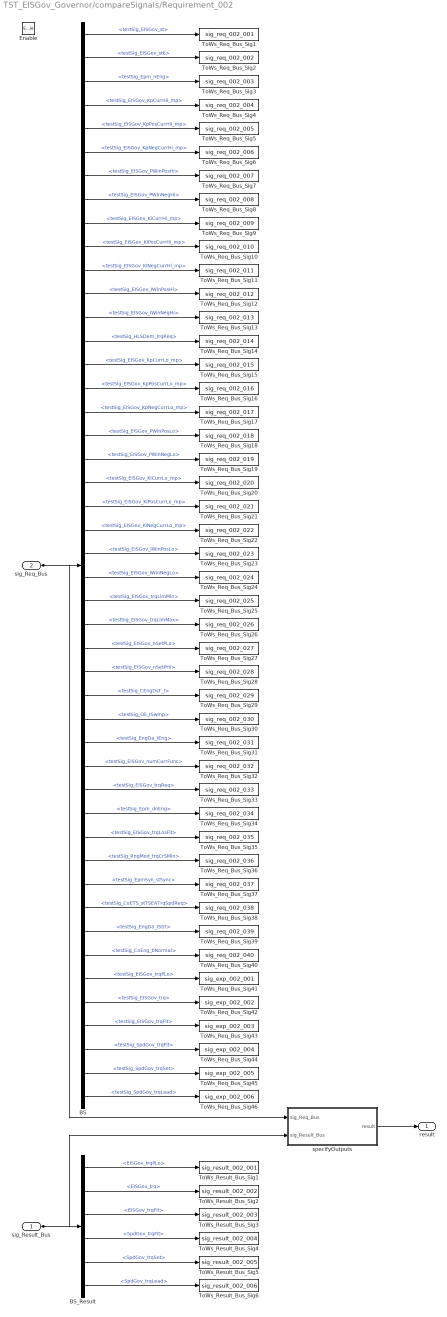
== system TST_EISGov_Governor/compareSignals/Requirement_002 ==
  sig_Result_Bus : Inport
  sig_Req_Bus : Inport  Port=2
  Enable : EnablePort
  BS : BusSelector  OutputSignals=testSig_EISGov_st,testSig_EISGov_st6,testSig_Epm_nEng,testSig_EISGov_KpCurrHi_mp,testSig_EISGov_KpPosCurrHi_mp,testSig_EISGov_KpNegCurrHi_mp,testSig_EISGov_PWinPosHi,testSig_EISGov_PWinNegHi,testSig_EISGov_KiCurrHi_mp,testSig_EISGov_KiPosCurrHi_mp,testSig_EISGov_KiNegCurrHi_mp,testSig_EISGov_IWinPosHi,testSig_EISGov_IWinNegHi,testSig_HLSDem_trqReq,testSig_EISGov_KpCurrLo_mp,testSig_EISGov_KpPosCurrLo_mp,testSig_EISGov_KpNegCurrLo_mp,testSig_EISGov_PWinPosLo,testSig_EISGov_PWinNegLo,testSig_EISGov_KiCurrLo_mp,testSig_EISGov_KiPosCurrLo_mp,testSig_EISGov_KiNegCurrLo_mp,testSig_EISGov_IWinPosLo,testSig_EISGov_IWinNegLo,testSig_EISGov_trqLimMin,testSig_EISGov_trqLimMax,testSig_EISGov_nSetPLo,testSig_EISGov_nSetPHi,testSig_CEngDsT_t,testSig_Oil_tSwmp,testSig_EngDa_tEng,testSig_EISGov_numCurrFunc,testSig_EISGov_trqReq,testSig_Epm_dnEng,testSig_EISGov_trqLosFlt,testSig_RngMod_trqCrSMin,testSig_EpmSyn_stSync,testSig_CoETS_stTSEATrqSpdReq,testSig_EngDa_tStrt,testSig_CoEng_tiNormal,testSig_EISGov_trqPLo,testSig_EISGov_trq,testSig_EISGov_trqFlt,testSig_SpdGov_trqFlt,testSig_SpdGov_trqSet,testSig_SpdGov_trqLead
  BS_Result : BusSelector  OutputSignals=EISGov_trqPLo,EISGov_trq,EISGov_trqFlt,SpdGov_trqFlt,SpdGov_trqSet,SpdGov_trqLead
  ToWs_Req_Bus_Sig1 : ToWorkspace  VariableName=sig_req_002_001  SaveFormat=Structure With Time
  ToWs_Req_Bus_Sig10 : ToWorkspace  VariableName=sig_req_002_010  SaveFormat=Structure With Time
  ToWs_Req_Bus_Sig11 : ToWorkspace  VariableName=sig_req_002_011  SaveFormat=Structure With Time
  ToWs_Req_Bus_Sig12 : ToWorkspace  VariableName=sig_req_002_012  SaveFormat=Structure With Time
  ToWs_Req_Bus_Sig13 : ToWorkspace  VariableName=sig_req_002_013  SaveFormat=Structure With Time
  ToWs_Req_Bus_Sig14 : ToWorkspace  VariableName=sig_req_002_014  SaveFormat=Structure With Time
  ToWs_Req_Bus_Sig15 : ToWorkspace  VariableName=sig_req_002_015  SaveFormat=Structure With Time
  ToWs_Req_Bus_Sig16 : ToWorkspace  VariableName=sig_req_002_016  SaveFormat=Structure With Time
  ToWs_Req_Bus_Sig17 : ToWorkspace  VariableName=sig_req_002_017  SaveFormat=Structure With Time
  ToWs_Req_Bus_Sig18 : ToWorkspace  VariableName=sig_req_002_018  SaveFormat=Structure With Time
  ToWs_Req_Bus_Sig19 : ToWorkspace  VariableName=sig_req_002_019  SaveFormat=Structure With Time
  ToWs_Req_Bus_Sig2 : ToWorkspace  VariableName=sig_req_002_002  SaveFormat=Structure With Time
  ToWs_Req_Bus_Sig20 : ToWorkspace  VariableName=sig_req_002_020  SaveFormat=Structure With Time
  ToWs_Req_Bus_Sig21 : ToWorkspace  VariableName=sig_req_002_021  SaveFormat=Structure With Time
  ToWs_Req_Bus_Sig22 : ToWorkspace  VariableName=sig_req_002_022  SaveFormat=Structure With Time
  ToWs_Req_Bus_Sig23 : ToWorkspace  VariableName=sig_req_002_023  SaveFormat=Structure With Time
  ToWs_Req_Bus_Sig24 : ToWorkspace  VariableName=sig_req_002_024  SaveFormat=Structure With Time
  ToWs_Req_Bus_Sig25 : ToWorkspace  VariableName=sig_req_002_025  SaveFormat=Structure With Time
  ToWs_Req_Bus_Sig26 : ToWorkspace  VariableName=sig_req_002_026  SaveFormat=Structure With Time
  ToWs_Req_Bus_Sig27 : ToWorkspace  VariableName=sig_req_002_027  SaveFormat=Structure With Time
  ToWs_Req_Bus_Sig28 : ToWorkspace  VariableName=sig_req_002_028  SaveFormat=Structure With Time
  ToWs_Req_Bus_Sig29 : ToWorkspace  VariableName=sig_req_002_029  SaveFormat=Structure With Time
  ToWs_Req_Bus_Sig3 : ToWorkspace  VariableName=sig_req_002_003  SaveFormat=Structure With Time
  ToWs_Req_Bus_Sig30 : ToWorkspace  VariableName=sig_req_002_030  SaveFormat=Structure With Time
  ToWs_Req_Bus_Sig31 : ToWorkspace  VariableName=sig_req_002_031  SaveFormat=Structure With Time
  ToWs_Req_Bus_Sig32 : ToWorkspace  VariableName=sig_req_002_032  SaveFormat=Structure With Time
  ToWs_Req_Bus_Sig33 : ToWorkspace  VariableName=sig_req_002_033  SaveFormat=Structure With Time
  ToWs_Req_Bus_Sig34 : ToWorkspace  VariableName=sig_req_002_034  SaveFormat=Structure With Time
  ToWs_Req_Bus_Sig35 : ToWorkspace  VariableName=sig_req_002_035  SaveFormat=Structure With Time
  ToWs_Req_Bus_Sig36 : ToWorkspace  VariableName=sig_req_002_036  SaveFormat=Structure With Time
  ToWs_Req_Bus_Sig37 : ToWorkspace  VariableName=sig_req_002_037  SaveFormat=Structure With Time
  ToWs_Req_Bus_Sig38 : ToWorkspace  VariableName=sig_req_002_038  SaveFormat=Structure With Time
  ToWs_Req_Bus_Sig39 : ToWorkspace  VariableName=sig_req_002_039  SaveFormat=Structure With Time
  ToWs_Req_Bus_Sig4 : ToWorkspace  VariableName=sig_req_002_004  SaveFormat=Structure With Time
  ToWs_Req_Bus_Sig40 : ToWorkspace  VariableName=sig_req_002_040  SaveFormat=Structure With Time
  ToWs_Req_Bus_Sig41 : ToWorkspace  VariableName=sig_exp_002_001  SaveFormat=Structure With Time
  ToWs_Req_Bus_Sig42 : ToWorkspace  VariableName=sig_exp_002_002  SaveFormat=Structure With Time
  ToWs_Req_Bus_Sig43 : ToWorkspace  VariableName=sig_exp_002_003  SaveFormat=Structure With Time
  ToWs_Req_Bus_Sig44 : ToWorkspace  VariableName=sig_exp_002_004  SaveFormat=Structure With Time
  ToWs_Req_Bus_Sig45 : ToWorkspace  VariableName=sig_exp_002_005  SaveFormat=Structure With Time
  ToWs_Req_Bus_Sig46 : ToWorkspace  VariableName=sig_exp_002_006  SaveFormat=Structure With Time
  ToWs_Req_Bus_Sig5 : ToWorkspace  VariableName=sig_req_002_005  SaveFormat=Structure With Time
  ToWs_Req_Bus_Sig6 : ToWorkspace  VariableName=sig_req_002_006  SaveFormat=Structure With Time
  ToWs_Req_Bus_Sig7 : ToWorkspace  VariableName=sig_req_002_007  SaveFormat=Structure With Time
  ToWs_Req_Bus_Sig8 : ToWorkspace  VariableName=sig_req_002_008  SaveFormat=Structure With Time
  ToWs_Req_Bus_Sig9 : ToWorkspace  VariableName=sig_req_002_009  SaveFormat=Structure With Time
  ToWs_Result_Bus_Sig1 : ToWorkspace  VariableName=sig_result_002_001  SaveFormat=Structure With Time
  ToWs_Result_Bus_Sig2 : ToWorkspace  VariableName=sig_result_002_002  SaveFormat=Structure With Time
  ToWs_Result_Bus_Sig3 : ToWorkspace  VariableName=sig_result_002_003  SaveFormat=Structure With Time
  ToWs_Result_Bus_Sig4 : ToWorkspace  VariableName=sig_result_002_004  SaveFormat=Structure With Time
  ToWs_Result_Bus_Sig5 : ToWorkspace  VariableName=sig_result_002_005  SaveFormat=Structure With Time
  ToWs_Result_Bus_Sig6 : ToWorkspace  VariableName=sig_result_002_006  SaveFormat=Structure With Time
  specifyOutputs : Subsystem
  result : Outport
  wires:
  sig_Req_Bus/1 -> BS/1, specifyOutputs/1(sig_Req_Bus)
  BS/1 -> ToWs_Req_Bus_Sig1/1  "<testSig_EISGov_st>"
  BS/2 -> ToWs_Req_Bus_Sig2/1  "<testSig_EISGov_st6>"
  BS/3 -> ToWs_Req_Bus_Sig3/1  "<testSig_Epm_nEng>"
  BS/4 -> ToWs_Req_Bus_Sig4/1  "<testSig_EISGov_KpCurrHi_mp>"
  BS/5 -> ToWs_Req_Bus_Sig5/1  "<testSig_EISGov_KpPosCurrHi_mp>"
  BS/6 -> ToWs_Req_Bus_Sig6/1  "<testSig_EISGov_KpNegCurrHi_mp>"
  BS/7 -> ToWs_Req_Bus_Sig7/1  "<testSig_EISGov_PWinPosHi>"
  BS/8 -> ToWs_Req_Bus_Sig8/1  "<testSig_EISGov_PWinNegHi>"
  BS/9 -> ToWs_Req_Bus_Sig9/1  "<testSig_EISGov_KiCurrHi_mp>"
  BS/10 -> ToWs_Req_Bus_Sig10/1  "<testSig_EISGov_KiPosCurrHi_mp>"
  BS/11 -> ToWs_Req_Bus_Sig11/1  "<testSig_EISGov_KiNegCurrHi_mp>"
  BS/12 -> ToWs_Req_Bus_Sig12/1  "<testSig_EISGov_IWinPosHi>"
  BS/13 -> ToWs_Req_Bus_Sig13/1  "<testSig_EISGov_IWinNegHi>"
  BS/14 -> ToWs_Req_Bus_Sig14/1  "<testSig_HLSDem_trqReq>"
  BS/15 -> ToWs_Req_Bus_Sig15/1  "<testSig_EISGov_KpCurrLo_mp>"
  BS/16 -> ToWs_Req_Bus_Sig16/1  "<testSig_EISGov_KpPosCurrLo_mp>"
  BS/17 -> ToWs_Req_Bus_Sig17/1  "<testSig_EISGov_KpNegCurrLo_mp>"
  BS/18 -> ToWs_Req_Bus_Sig18/1  "<testSig_EISGov_PWinPosLo>"
  BS/19 -> ToWs_Req_Bus_Sig19/1  "<testSig_EISGov_PWinNegLo>"
  BS/20 -> ToWs_Req_Bus_Sig20/1  "<testSig_EISGov_KiCurrLo_mp>"
  BS/21 -> ToWs_Req_Bus_Sig21/1  "<testSig_EISGov_KiPosCurrLo_mp>"
  BS/22 -> ToWs_Req_Bus_Sig22/1  "<testSig_EISGov_KiNegCurrLo_mp>"
  BS/23 -> ToWs_Req_Bus_Sig23/1  "<testSig_EISGov_IWinPosLo>"
  BS/24 -> ToWs_Req_Bus_Sig24/1  "<testSig_EISGov_IWinNegLo>"
  BS/25 -> ToWs_Req_Bus_Sig25/1  "<testSig_EISGov_trqLimMin>"
  BS/26 -> ToWs_Req_Bus_Sig26/1  "<testSig_EISGov_trqLimMax>"
  BS/27 -> ToWs_Req_Bus_Sig27/1  "<testSig_EISGov_nSetPLo>"
  BS/28 -> ToWs_Req_Bus_Sig28/1  "<testSig_EISGov_nSetPHi>"
  BS/29 -> ToWs_Req_Bus_Sig29/1  "<testSig_CEngDsT_t>"
  BS/30 -> ToWs_Req_Bus_Sig30/1  "<testSig_Oil_tSwmp>"
  BS/31 -> ToWs_Req_Bus_Sig31/1  "<testSig_EngDa_tEng>"
  BS/32 -> ToWs_Req_Bus_Sig32/1  "<testSig_EISGov_numCurrFunc>"
  BS/33 -> ToWs_Req_Bus_Sig33/1  "<testSig_EISGov_trqReq>"
  BS/34 -> ToWs_Req_Bus_Sig34/1  "<testSig_Epm_dnEng>"
  BS/35 -> ToWs_Req_Bus_Sig35/1  "<testSig_EISGov_trqLosFlt>"
  BS/36 -> ToWs_Req_Bus_Sig36/1  "<testSig_RngMod_trqCrSMin>"
  BS/37 -> ToWs_Req_Bus_Sig37/1  "<testSig_EpmSyn_stSync>"
  BS/38 -> ToWs_Req_Bus_Sig38/1  "<testSig_CoETS_stTSEATrqSpdReq>"
  BS/39 -> ToWs_Req_Bus_Sig39/1  "<testSig_EngDa_tStrt>"
  BS/40 -> ToWs_Req_Bus_Sig40/1  "<testSig_CoEng_tiNormal>"
  BS/41 -> ToWs_Req_Bus_Sig41/1  "<testSig_EISGov_trqPLo>"
  BS/42 -> ToWs_Req_Bus_Sig42/1  "<testSig_EISGov_trq>"
  BS/43 -> ToWs_Req_Bus_Sig43/1  "<testSig_EISGov_trqFlt>"
  BS/44 -> ToWs_Req_Bus_Sig44/1  "<testSig_SpdGov_trqFlt>"
  BS/45 -> ToWs_Req_Bus_Sig45/1  "<testSig_SpdGov_trqSet>"
  BS/46 -> ToWs_Req_Bus_Sig46/1  "<testSig_SpdGov_trqLead>"
  sig_Result_Bus/1 -> BS_Result/1, specifyOutputs/2(sig_Result_Bus)
  BS_Result/1 -> ToWs_Result_Bus_Sig1/1  "<EISGov_trqPLo>"
  BS_Result/2 -> ToWs_Result_Bus_Sig2/1  "<EISGov_trq>"
  BS_Result/3 -> ToWs_Result_Bus_Sig3/1  "<EISGov_trqFlt>"
  BS_Result/4 -> ToWs_Result_Bus_Sig4/1  "<SpdGov_trqFlt>"
  BS_Result/5 -> ToWs_Result_Bus_Sig5/1  "<SpdGov_trqSet>"
  BS_Result/6 -> ToWs_Result_Bus_Sig6/1  "<SpdGov_trqLead>"
  specifyOutputs/1(result) -> result/1

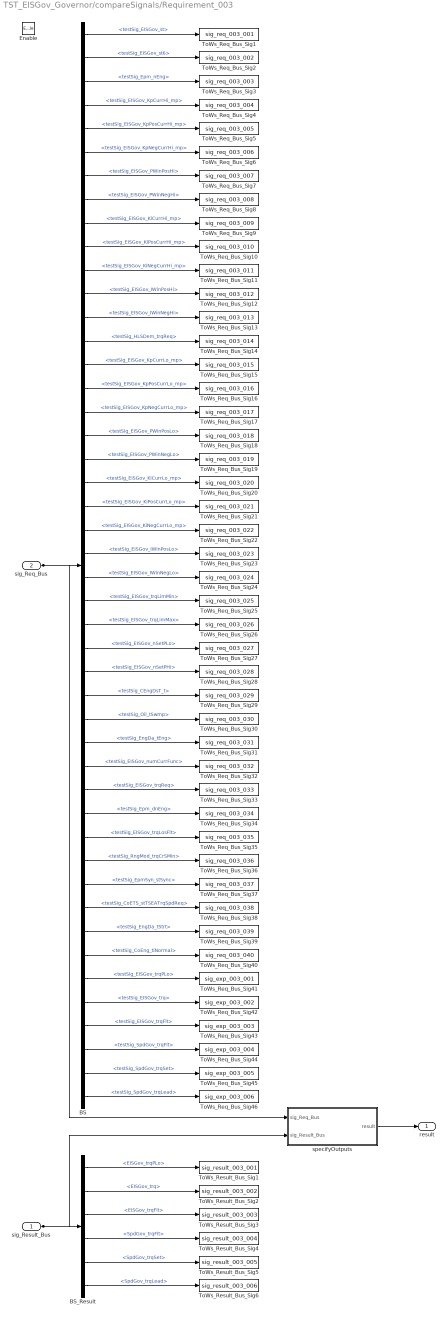
== system TST_EISGov_Governor/compareSignals/Requirement_003 ==
  sig_Result_Bus : Inport
  sig_Req_Bus : Inport  Port=2
  Enable : EnablePort
  BS : BusSelector  OutputSignals=testSig_EISGov_st,testSig_EISGov_st6,testSig_Epm_nEng,testSig_EISGov_KpCurrHi_mp,testSig_EISGov_KpPosCurrHi_mp,testSig_EISGov_KpNegCurrHi_mp,testSig_EISGov_PWinPosHi,testSig_EISGov_PWinNegHi,testSig_EISGov_KiCurrHi_mp,testSig_EISGov_KiPosCurrHi_mp,testSig_EISGov_KiNegCurrHi_mp,testSig_EISGov_IWinPosHi,testSig_EISGov_IWinNegHi,testSig_HLSDem_trqReq,testSig_EISGov_KpCurrLo_mp,testSig_EISGov_KpPosCurrLo_mp,testSig_EISGov_KpNegCurrLo_mp,testSig_EISGov_PWinPosLo,testSig_EISGov_PWinNegLo,testSig_EISGov_KiCurrLo_mp,testSig_EISGov_KiPosCurrLo_mp,testSig_EISGov_KiNegCurrLo_mp,testSig_EISGov_IWinPosLo,testSig_EISGov_IWinNegLo,testSig_EISGov_trqLimMin,testSig_EISGov_trqLimMax,testSig_EISGov_nSetPLo,testSig_EISGov_nSetPHi,testSig_CEngDsT_t,testSig_Oil_tSwmp,testSig_EngDa_tEng,testSig_EISGov_numCurrFunc,testSig_EISGov_trqReq,testSig_Epm_dnEng,testSig_EISGov_trqLosFlt,testSig_RngMod_trqCrSMin,testSig_EpmSyn_stSync,testSig_CoETS_stTSEATrqSpdReq,testSig_EngDa_tStrt,testSig_CoEng_tiNormal,testSig_EISGov_trqPLo,testSig_EISGov_trq,testSig_EISGov_trqFlt,testSig_SpdGov_trqFlt,testSig_SpdGov_trqSet,testSig_SpdGov_trqLead
  BS_Result : BusSelector  OutputSignals=EISGov_trqPLo,EISGov_trq,EISGov_trqFlt,SpdGov_trqFlt,SpdGov_trqSet,SpdGov_trqLead
  ToWs_Req_Bus_Sig1 : ToWorkspace  VariableName=sig_req_003_001  SaveFormat=Structure With Time
  ToWs_Req_Bus_Sig10 : ToWorkspace  VariableName=sig_req_003_010  SaveFormat=Structure With Time
  ToWs_Req_Bus_Sig11 : ToWorkspace  VariableName=sig_req_003_011  SaveFormat=Structure With Time
  ToWs_Req_Bus_Sig12 : ToWorkspace  VariableName=sig_req_003_012  SaveFormat=Structure With Time
  ToWs_Req_Bus_Sig13 : ToWorkspace  VariableName=sig_req_003_013  SaveFormat=Structure With Time
  ToWs_Req_Bus_Sig14 : ToWorkspace  VariableName=sig_req_003_014  SaveFormat=Structure With Time
  ToWs_Req_Bus_Sig15 : ToWorkspace  VariableName=sig_req_003_015  SaveFormat=Structure With Time
  ToWs_Req_Bus_Sig16 : ToWorkspace  VariableName=sig_req_003_016  SaveFormat=Structure With Time
  ToWs_Req_Bus_Sig17 : ToWorkspace  VariableName=sig_req_003_017  SaveFormat=Structure With Time
  ToWs_Req_Bus_Sig18 : ToWorkspace  VariableName=sig_req_003_018  SaveFormat=Structure With Time
  ToWs_Req_Bus_Sig19 : ToWorkspace  VariableName=sig_req_003_019  SaveFormat=Structure With Time
  ToWs_Req_Bus_Sig2 : ToWorkspace  VariableName=sig_req_003_002  SaveFormat=Structure With Time
  ToWs_Req_Bus_Sig20 : ToWorkspace  VariableName=sig_req_003_020  SaveFormat=Structure With Time
  ToWs_Req_Bus_Sig21 : ToWorkspace  VariableName=sig_req_003_021  SaveFormat=Structure With Time
  ToWs_Req_Bus_Sig22 : ToWorkspace  VariableName=sig_req_003_022  SaveFormat=Structure With Time
  ToWs_Req_Bus_Sig23 : ToWorkspace  VariableName=sig_req_003_023  SaveFormat=Structure With Time
  ToWs_Req_Bus_Sig24 : ToWorkspace  VariableName=sig_req_003_024  SaveFormat=Structure With Time
  ToWs_Req_Bus_Sig25 : ToWorkspace  VariableName=sig_req_003_025  SaveFormat=Structure With Time
  ToWs_Req_Bus_Sig26 : ToWorkspace  VariableName=sig_req_003_026  SaveFormat=Structure With Time
  ToWs_Req_Bus_Sig27 : ToWorkspace  VariableName=sig_req_003_027  SaveFormat=Structure With Time
  ToWs_Req_Bus_Sig28 : ToWorkspace  VariableName=sig_req_003_028  SaveFormat=Structure With Time
  ToWs_Req_Bus_Sig29 : ToWorkspace  VariableName=sig_req_003_029  SaveFormat=Structure With Time
  ToWs_Req_Bus_Sig3 : ToWorkspace  VariableName=sig_req_003_003  SaveFormat=Structure With Time
  ToWs_Req_Bus_Sig30 : ToWorkspace  VariableName=sig_req_003_030  SaveFormat=Structure With Time
  ToWs_Req_Bus_Sig31 : ToWorkspace  VariableName=sig_req_003_031  SaveFormat=Structure With Time
  ToWs_Req_Bus_Sig32 : ToWorkspace  VariableName=sig_req_003_032  SaveFormat=Structure With Time
  ToWs_Req_Bus_Sig33 : ToWorkspace  VariableName=sig_req_003_033  SaveFormat=Structure With Time
  ToWs_Req_Bus_Sig34 : ToWorkspace  VariableName=sig_req_003_034  SaveFormat=Structure With Time
  ToWs_Req_Bus_Sig35 : ToWorkspace  VariableName=sig_req_003_035  SaveFormat=Structure With Time
  ToWs_Req_Bus_Sig36 : ToWorkspace  VariableName=sig_req_003_036  SaveFormat=Structure With Time
  ToWs_Req_Bus_Sig37 : ToWorkspace  VariableName=sig_req_003_037  SaveFormat=Structure With Time
  ToWs_Req_Bus_Sig38 : ToWorkspace  VariableName=sig_req_003_038  SaveFormat=Structure With Time
  ToWs_Req_Bus_Sig39 : ToWorkspace  VariableName=sig_req_003_039  SaveFormat=Structure With Time
  ToWs_Req_Bus_Sig4 : ToWorkspace  VariableName=sig_req_003_004  SaveFormat=Structure With Time
  ToWs_Req_Bus_Sig40 : ToWorkspace  VariableName=sig_req_003_040  SaveFormat=Structure With Time
  ToWs_Req_Bus_Sig41 : ToWorkspace  VariableName=sig_exp_003_001  SaveFormat=Structure With Time
  ToWs_Req_Bus_Sig42 : ToWorkspace  VariableName=sig_exp_003_002  SaveFormat=Structure With Time
  ToWs_Req_Bus_Sig43 : ToWorkspace  VariableName=sig_exp_003_003  SaveFormat=Structure With Time
  ToWs_Req_Bus_Sig44 : ToWorkspace  VariableName=sig_exp_003_004  SaveFormat=Structure With Time
  ToWs_Req_Bus_Sig45 : ToWorkspace  VariableName=sig_exp_003_005  SaveFormat=Structure With Time
  ToWs_Req_Bus_Sig46 : ToWorkspace  VariableName=sig_exp_003_006  SaveFormat=Structure With Time
  ToWs_Req_Bus_Sig5 : ToWorkspace  VariableName=sig_req_003_005  SaveFormat=Structure With Time
  ToWs_Req_Bus_Sig6 : ToWorkspace  VariableName=sig_req_003_006  SaveFormat=Structure With Time
  ToWs_Req_Bus_Sig7 : ToWorkspace  VariableName=sig_req_003_007  SaveFormat=Structure With Time
  ToWs_Req_Bus_Sig8 : ToWorkspace  VariableName=sig_req_003_008  SaveFormat=Structure With Time
  ToWs_Req_Bus_Sig9 : ToWorkspace  VariableName=sig_req_003_009  SaveFormat=Structure With Time
  ToWs_Result_Bus_Sig1 : ToWorkspace  VariableName=sig_result_003_001  SaveFormat=Structure With Time
  ToWs_Result_Bus_Sig2 : ToWorkspace  VariableName=sig_result_003_002  SaveFormat=Structure With Time
  ToWs_Result_Bus_Sig3 : ToWorkspace  VariableName=sig_result_003_003  SaveFormat=Structure With Time
  ToWs_Result_Bus_Sig4 : ToWorkspace  VariableName=sig_result_003_004  SaveFormat=Structure With Time
  ToWs_Result_Bus_Sig5 : ToWorkspace  VariableName=sig_result_003_005  SaveFormat=Structure With Time
  ToWs_Result_Bus_Sig6 : ToWorkspace  VariableName=sig_result_003_006  SaveFormat=Structure With Time
  specifyOutputs : Subsystem
  result : Outport
  wires:
  sig_Req_Bus/1 -> BS/1, specifyOutputs/1(sig_Req_Bus)
  BS/1 -> ToWs_Req_Bus_Sig1/1  "<testSig_EISGov_st>"
  BS/2 -> ToWs_Req_Bus_Sig2/1  "<testSig_EISGov_st6>"
  BS/3 -> ToWs_Req_Bus_Sig3/1  "<testSig_Epm_nEng>"
  BS/4 -> ToWs_Req_Bus_Sig4/1  "<testSig_EISGov_KpCurrHi_mp>"
  BS/5 -> ToWs_Req_Bus_Sig5/1  "<testSig_EISGov_KpPosCurrHi_mp>"
  BS/6 -> ToWs_Req_Bus_Sig6/1  "<testSig_EISGov_KpNegCurrHi_mp>"
  BS/7 -> ToWs_Req_Bus_Sig7/1  "<testSig_EISGov_PWinPosHi>"
  BS/8 -> ToWs_Req_Bus_Sig8/1  "<testSig_EISGov_PWinNegHi>"
  BS/9 -> ToWs_Req_Bus_Sig9/1  "<testSig_EISGov_KiCurrHi_mp>"
  BS/10 -> ToWs_Req_Bus_Sig10/1  "<testSig_EISGov_KiPosCurrHi_mp>"
  BS/11 -> ToWs_Req_Bus_Sig11/1  "<testSig_EISGov_KiNegCurrHi_mp>"
  BS/12 -> ToWs_Req_Bus_Sig12/1  "<testSig_EISGov_IWinPosHi>"
  BS/13 -> ToWs_Req_Bus_Sig13/1  "<testSig_EISGov_IWinNegHi>"
  BS/14 -> ToWs_Req_Bus_Sig14/1  "<testSig_HLSDem_trqReq>"
  BS/15 -> ToWs_Req_Bus_Sig15/1  "<testSig_EISGov_KpCurrLo_mp>"
  BS/16 -> ToWs_Req_Bus_Sig16/1  "<testSig_EISGov_KpPosCurrLo_mp>"
  BS/17 -> ToWs_Req_Bus_Sig17/1  "<testSig_EISGov_KpNegCurrLo_mp>"
  BS/18 -> ToWs_Req_Bus_Sig18/1  "<testSig_EISGov_PWinPosLo>"
  BS/19 -> ToWs_Req_Bus_Sig19/1  "<testSig_EISGov_PWinNegLo>"
  BS/20 -> ToWs_Req_Bus_Sig20/1  "<testSig_EISGov_KiCurrLo_mp>"
  BS/21 -> ToWs_Req_Bus_Sig21/1  "<testSig_EISGov_KiPosCurrLo_mp>"
  BS/22 -> ToWs_Req_Bus_Sig22/1  "<testSig_EISGov_KiNegCurrLo_mp>"
  BS/23 -> ToWs_Req_Bus_Sig23/1  "<testSig_EISGov_IWinPosLo>"
  BS/24 -> ToWs_Req_Bus_Sig24/1  "<testSig_EISGov_IWinNegLo>"
  BS/25 -> ToWs_Req_Bus_Sig25/1  "<testSig_EISGov_trqLimMin>"
  BS/26 -> ToWs_Req_Bus_Sig26/1  "<testSig_EISGov_trqLimMax>"
  BS/27 -> ToWs_Req_Bus_Sig27/1  "<testSig_EISGov_nSetPLo>"
  BS/28 -> ToWs_Req_Bus_Sig28/1  "<testSig_EISGov_nSetPHi>"
  BS/29 -> ToWs_Req_Bus_Sig29/1  "<testSig_CEngDsT_t>"
  BS/30 -> ToWs_Req_Bus_Sig30/1  "<testSig_Oil_tSwmp>"
  BS/31 -> ToWs_Req_Bus_Sig31/1  "<testSig_EngDa_tEng>"
  BS/32 -> ToWs_Req_Bus_Sig32/1  "<testSig_EISGov_numCurrFunc>"
  BS/33 -> ToWs_Req_Bus_Sig33/1  "<testSig_EISGov_trqReq>"
  BS/34 -> ToWs_Req_Bus_Sig34/1  "<testSig_Epm_dnEng>"
  BS/35 -> ToWs_Req_Bus_Sig35/1  "<testSig_EISGov_trqLosFlt>"
  BS/36 -> ToWs_Req_Bus_Sig36/1  "<testSig_RngMod_trqCrSMin>"
  BS/37 -> ToWs_Req_Bus_Sig37/1  "<testSig_EpmSyn_stSync>"
  BS/38 -> ToWs_Req_Bus_Sig38/1  "<testSig_CoETS_stTSEATrqSpdReq>"
  BS/39 -> ToWs_Req_Bus_Sig39/1  "<testSig_EngDa_tStrt>"
  BS/40 -> ToWs_Req_Bus_Sig40/1  "<testSig_CoEng_tiNormal>"
  BS/41 -> ToWs_Req_Bus_Sig41/1  "<testSig_EISGov_trqPLo>"
  BS/42 -> ToWs_Req_Bus_Sig42/1  "<testSig_EISGov_trq>"
  BS/43 -> ToWs_Req_Bus_Sig43/1  "<testSig_EISGov_trqFlt>"
  BS/44 -> ToWs_Req_Bus_Sig44/1  "<testSig_SpdGov_trqFlt>"
  BS/45 -> ToWs_Req_Bus_Sig45/1  "<testSig_SpdGov_trqSet>"
  BS/46 -> ToWs_Req_Bus_Sig46/1  "<testSig_SpdGov_trqLead>"
  sig_Result_Bus/1 -> BS_Result/1, specifyOutputs/2(sig_Result_Bus)
  BS_Result/1 -> ToWs_Result_Bus_Sig1/1  "<EISGov_trqPLo>"
  BS_Result/2 -> ToWs_Result_Bus_Sig2/1  "<EISGov_trq>"
  BS_Result/3 -> ToWs_Result_Bus_Sig3/1  "<EISGov_trqFlt>"
  BS_Result/4 -> ToWs_Result_Bus_Sig4/1  "<SpdGov_trqFlt>"
  BS_Result/5 -> ToWs_Result_Bus_Sig5/1  "<SpdGov_trqSet>"
  BS_Result/6 -> ToWs_Result_Bus_Sig6/1  "<SpdGov_trqLead>"
  specifyOutputs/1(result) -> result/1
